simulink model "quadripulse_controller16"  (R2016a)
settings: Solver=FixedStepAuto  StartTime=0.0  StopTime=Inf  RelTol=1e-3
values from neighbouring files (symbols this model uses):
  amplitudeinterval = [0 10000]    [PIP_SetVariables4Compilation.m]
  amplitudeinterval_percentiles = [0.25 0.75]    [PIP_SetVariables4Compilation.m]
  closedloopmode = 0    [PIP_SetVariables4Compilation.m]
  fft_bin_indices_zero_based = [8 13]    [PIP_SetVariables4Compilation.m]
  fir_filter_coefficients = get(design(fdesign.bandpass('n,fst1,fp1,fp2,fst2', 128, 4, 8, 12, 16, 1000), 'firls', 'FilterStructure', 'dffirt'), 'Numerator')    [PIP_SetVariables4Compilation.m]
  forecast_offset_ms = 0    [PIP_SetVariables4Compilation.m]
  marker_id = 0    [PIP_SetVariables4Compilation.m]
  phasecondition = 1    [PIP_SetVariables4Compilation.m]
  reset = 0    [PIP_SetVariables4Compilation.m]
  spatial_filter = zeros(1,N); spatial_filter(chan_center) = 1; spatial_filter(chan_surround) = -1/length(chan_surround)    [PIP_SetVariables4Compilation.m]
  timeinsecondsandtriggerchannel = [0,1;0.1,2]    [PIP_SetVariables4Compilation.m]
undefined symbols (not defined in the file or in its folder): a, b, Columns, MF, PD2, Radix, Rows
libraries: dspmtrx3 x11, slrtlib x10, simulink x9, dspstat3 x5, dspsigops x4, commsequence2 x1, dspobslib x1, dspspect3 x1, dspfdesign x1, xpcueilib x1, xpcparallelportlib x1, xpciplib x1
settings Model: SimulationMode=external  Creator=BNP Lab User  LastModifiedBy=BNP Lab
settings SolverCC: EnableConcurrentExecution=on
settings DataIOCC: LimitDataPoints=on  SaveFormat=StructureWithTime  SaveOutput=off  SignalLogging=off  DSMLogging=off  SaveTime=off
settings OptimizationCC: BlockReduction=off  OptimizeBlockIOStorage=off  BufferReuse=off  GlobalBufferReuse=off  ExpressionFolding=off  LocalBlockOutputs=off
settings DebuggingCC: AllowSymbolicDim=off
settings HardwareCC: ProdBitPerPointer=32  ProdLargestAtomicFloat=None  ProdWordSize=32  ProdHWDeviceType=Generic->32-bit x86 compatible
settings ModelReferenceCC: PropagateSignalLabelsOutOfModel=off
settings RTWCC: SystemTargetFile=slrt.tlc  TemplateMakefile=slrt_default_tmf  Description=Simulink Real-Time  RTWCompilerOptimization=on

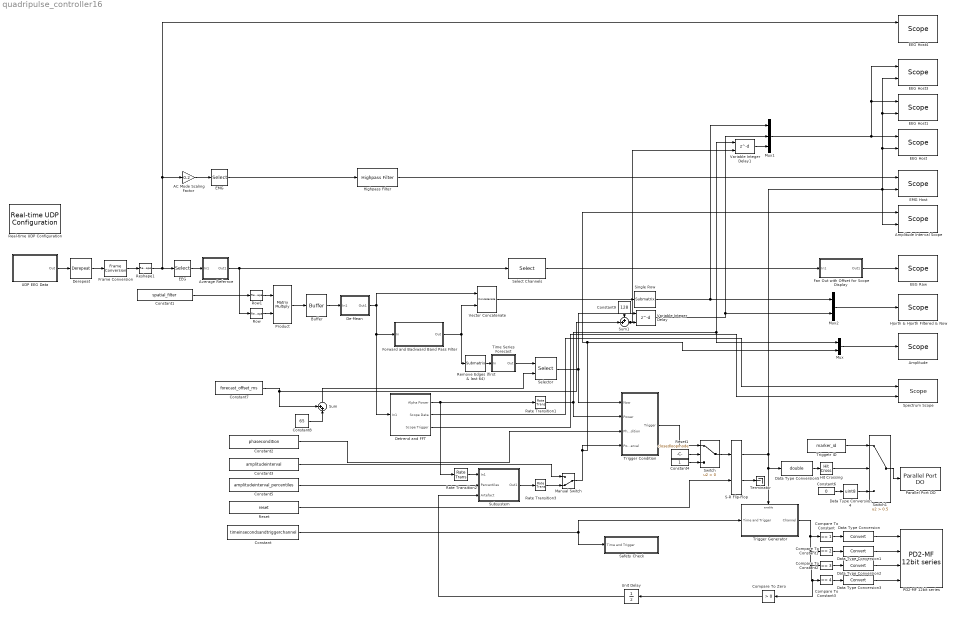
== system quadripulse_controller16 ==
  " Amplitude" : slrtlib/Displays and Logging/Scope   scopeno=3  scopetype=Target  autostart=on  viewmode=Graphical sliding  formatstr='%15.6f'  grid=on  ylimits=[0,0]  nosamples=100  noprepostsamples=0  interleave=100  triggermode=FreeRun  triggersignal=1  trigsignalfromport=on  triggerlevel=0.5  triggerslope=Rising  triggerscope=1  triggersample=0  filename=data.dat  mode=Lazy  writesize=512  autorestart=off  dynamicfilemode=off  maxwritefilesize=512*1024^2
  AC Mode Scaling Factor : Gain  Gain=0.2
  Amplitude Interval Scope : slrtlib/Displays and Logging/Scope   scopeno=10  scopetype=Host  autostart=on  viewmode=Graphical redraw  formatstr='%15.6f'  grid=on  ylimits=[0,0]  nosamples=3  noprepostsamples=-2  interleave=1  triggermode=Signal triggering  triggersignal=1  trigsignalfromport=on  triggerlevel=0.5  triggerslope=Rising  triggerscope=1  triggersample=0  filename=data.dat  mode=Lazy  writesize=512  autorestart=off  dynamicfilemode=off  maxwritefilesize=512*1024^2
  Average Refernce : Subsystem
  Buffer : Buffer  N=512  V=511  TreatMby1Signals=One channel  OutputFrames=off
  Compare To Constant : simulink/Logic and Bit Operations/Compare To Constant  relop===  const=1  OutDataTypeStr=boolean
  Compare To Constant1 : simulink/Logic and Bit Operations/Compare To Constant  relop===  const=2  OutDataTypeStr=boolean
  Compare To Constant2 : simulink/Logic and Bit Operations/Compare To Constant  relop===  const=3  OutDataTypeStr=boolean
  Compare To Constant3 : simulink/Logic and Bit Operations/Compare To Constant  relop===  const=4  OutDataTypeStr=boolean
  Compare To Zero : simulink/Logic and Bit Operations/Compare To Zero  relop=>  OutDataTypeStr=boolean
  Constant : Constant  Value=timeinsecondsandtriggerchannel  OutDataTypeStr=double  SampleTime=-1
  Constant1 : Constant  Value=spatial_filter  SampleTime=-1
  Constant2 : Constant  Value=phasecondition  SampleTime=-1
  Constant3 : Constant  Value=amplitudeinterval  SampleTime=-1
  Constant4 : Constant  OutDataTypeStr=boolean
  Constant5 : Constant  Value=amplitudeinterval_percentiles  SampleTime=-1
  Constant6 : Constant  Value=0  OutDataTypeStr=boolean
  Constant7 : Constant  Value=forecast_offset_ms  SampleTime=-1
  Constant8 : Constant  Value=65
  Constant9 : Constant  Value=128
  Data Type Conversion{,1..3} (4 alike) : DataTypeConversion
  Data Type Conversion4 : DataTypeConversion  OutDataTypeStr=uint8
  Data Type Conversion5 : DataTypeConversion  OutDataTypeStr=double
  De-Mean : Subsystem
  Derepeat : commsequence2/Derepeat  N=5  mode=Unused parameter value  InputProcessing=Columns as channels (frame based)  RateOptions=Enforce single-rate processing  ic=0
  Detrend and FFT : Subsystem
  EEG : Selector  InputPortWidth=66  IndexOptions=Index vector (dialog)  Indices=1:64  OutputSizes=1
  EEG Host : slrtlib/Displays and Logging/Scope   scopeno=12  scopetype=Host  autostart=on  viewmode=Graphical redraw  formatstr='%15.6f'  grid=on  ylimits=[0,0]  nosamples=3000  noprepostsamples=-3000  interleave=1  triggermode=Signal triggering  triggersignal=1  trigsignalfromport=on  triggerlevel=0.5  triggerslope=Rising  triggerscope=1  triggersample=0  filename=data.dat  mode=Lazy  writesize=512  autorestart=off  dynamicfilemode=off  maxwritefilesize=512*1024^2
  EEG Host1 : slrtlib/Displays and Logging/Scope   scopeno=13  scopetype=Host  autostart=on  viewmode=Graphical redraw  formatstr='%15.6f'  grid=on  ylimits=[0,0]  nosamples=2000  noprepostsamples=-1000+128  interleave=1  triggermode=Signal triggering  triggersignal=1  trigsignalfromport=on  triggerlevel=0.5  triggerslope=Rising  triggerscope=1  triggersample=0  filename=data.dat  mode=Lazy  writesize=512  autorestart=off  dynamicfilemode=off  maxwritefilesize=512*1024^2
  EEG Host3 : slrtlib/Displays and Logging/Scope   scopeno=14  scopetype=Host  autostart=on  viewmode=Graphical redraw  formatstr='%15.6f'  grid=on  ylimits=[0,0]  nosamples=150  noprepostsamples=-50+128  interleave=1  triggermode=Signal triggering  triggersignal=1  trigsignalfromport=on  triggerlevel=0.5  triggerslope=Rising  triggerscope=1  triggersample=0  filename=data.dat  mode=Lazy  writesize=512  autorestart=off  dynamicfilemode=off  maxwritefilesize=512*1024^2
  EEG Host4 : slrtlib/Displays and Logging/Scope   scopeno=15  scopetype=Host  autostart=on  viewmode=Graphical redraw  formatstr='%15.6f'  grid=on  ylimits=[0,0]  nosamples=2000  noprepostsamples=-1000  interleave=1  triggermode=Signal triggering  triggersignal=1  trigsignalfromport=on  triggerlevel=0.5  triggerslope=Rising  triggerscope=1  triggersample=0  filename=data.dat  mode=Lazy  writesize=512  autorestart=off  dynamicfilemode=off  maxwritefilesize=512*1024^2
  EEG Raw : slrtlib/Displays and Logging/Scope   scopeno=1  scopetype=Target  autostart=on  viewmode=Graphical redraw  formatstr='%15.6f'  grid=on  ylimits=[0,0]  nosamples=500  noprepostsamples=-250  interleave=1  triggermode=FreeRun  triggersignal=1  trigsignalfromport=on  triggerlevel=0.5  triggerslope=Rising  triggerscope=1  triggersample=0  filename=data.dat  mode=Lazy  writesize=512  autorestart=off  dynamicfilemode=off  maxwritefilesize=512*1024^2
  EMG : Selector  InputPortWidth=66  IndexOptions=Index vector (dialog)  Indices=[65 66]  OutputSizes=1
  "EMG Host " : slrtlib/Displays and Logging/Scope   scopeno=11  scopetype=Host  autostart=on  viewmode=Graphical redraw  formatstr='%15.6f'  grid=on  ylimits=[0,0]  nosamples=150  noprepostsamples=50  interleave=1  triggermode=Signal triggering  triggersignal=1  trigsignalfromport=on  triggerlevel=0.5  triggerslope=Rising  triggerscope=1  triggersample=0  filename=data.dat  mode=Lazy  writesize=512  autorestart=off  dynamicfilemode=off  maxwritefilesize=512*1024^2
  "Fan Out with Offset for Scope Display " : Subsystem
  Forward and Backward Band Pass Filter : Subsystem
  Frame Conversion : FrameConversion  InheritSamplingMode=off  OutFrame=Sample-based
  Highpass Filter : dspfdesign/Highpass Filter  FilterType=FIR  DesignForMinimumOrder=off  FilterOrder=200  StopbandFrequency=8e3  PassbandFrequency=10  StopbandAttenuation=80  PassbandRipple=0.1  InheritSampleRate=off  SampleRate=1000  roundingMode=Floor  coeffsDataTypeStr=fixdt(1,16)  SimulateUsing=Interpreted execution
  Hit Crossing : HitCross  HitCrossingOffset=0.5  HitCrossingDirection=rising
  Hjorth & Hjorth Filtered & Now : slrtlib/Displays and Logging/Scope   scopeno=2  scopetype=Target  autostart=on  viewmode=Graphical redraw  formatstr='%15.6f'  grid=on  ylimits=[-0,0]  nosamples=500  noprepostsamples=-250+128  interleave=1  triggermode=FreeRun  triggersignal=1  trigsignalfromport=on  triggerlevel=0.5  triggerslope=Rising  triggerscope=1  triggersample=0  filename=data.dat  mode=Lazy  writesize=512  autorestart=off  dynamicfilemode=off  maxwritefilesize=512*1024^2
  Manual Switch : ManualSwitch  CurrentSetting=0
  Mux : Mux  Inputs=2
  Mux1 : Mux  Inputs=3
  Mux2 : Mux  Inputs=2
  PD2-MF 12bit series : xpcueilib/Digital Output/PD2-MF 12bit series  boardtypein=PD2-MF-64-3M/12H  channel=[1 2 3 4]  reset=[1 1 1 1]  initValue=[0 0 0 0]  sampletime=0.001  pcislot=-1
  "Parallel Port DO " : xpcparallelportlib/Digital Output/Parallel Port DO   BaseMask=Other  BaseString=0xc010  Format=Single 8-bit Port  Channels=[1]  InitialValues=[0]  FinalActions=[0]  FinalValues=[0]  SampleTime=0.001  Mode=1
  Product : Product  Multiplication=Matrix(*)
  Rate Transition1 : RateTransition  Integrity=off  OutPortSampleTimeOpt=Inherit  OutPortSampleTime=10
  Rate Transition2 : RateTransition  Integrity=off  OutPortSampleTime=0.1
  Rate Transition3 : RateTransition  Integrity=off  OutPortSampleTimeOpt=Inherit  OutPortSampleTime=0.1
  Real-time UDP Configuration : xpciplib/Real-time UDP  Configuration   ID=1  IpAddress=192.168.200.240  SubnetMask=255.255.255.0  Gateway=0.0.0.0  EthDrv=Intel Gigabit  PciBus=3  PciSlot=0  udpID=0  MulticastList=[]  Multicast={}
  Remove Edges (first & last 64) : dspmtrx3/Submatrix  RowSpan=Range of rows  RowStartMode=Index  RowStartIndex=65  RowEndMode=Offset from last  RowEndIndex=64  ColSpan=All columns  ColStartMode=First  ColStartIndex=1  ColEndMode=Offset from last  ColEndIndex=20
  Reset : Constant  Value=reset  OutDataTypeStr=boolean  SampleTime=0.001
  Reset1 : Constant  Value=closedloopmode  OutDataTypeStr=boolean  SampleTime=0.001
  Reshape1 : Reshape  OutputDimensionality=Row vector (2-D)
  Row : Reshape  OutputDimensionality=Column vector (2-D)
  Row1 : Reshape  OutputDimensionality=Row vector (2-D)
  S-R Flip-Flop : simulink_extras/Flip Flops/S-R Flip-Flop  initial_condition=0
  Safety Check : Subsystem
  Select Channels : Selector  InputPortWidth=65  IndexOptions=Index vector (dialog)  Indices=[5 21 23 25 27]  OutputSizes=1
  Selector : Selector  InputPortWidth=128  IndexOptions=Index vector (port)  Indices=forecast_offset_ms  OutputSizes=1
  Single Row : dspmtrx3/Submatrix  RowSpan=One row  RowStartMode=Offset from last  RowStartIndex=128  RowEndMode=Last  RowEndIndex=1  ColSpan=All columns  ColStartMode=Index  ColStartIndex=1  ColEndMode=Last  ColEndIndex=1
  "Spectrum Scope " : slrtlib/Displays and Logging/Scope   scopeno=4  scopetype=Target  autostart=on  viewmode=Graphical redraw  formatstr='%15.6f'  grid=on  ylimits=[0,0]  nosamples=100  noprepostsamples=0  interleave=1  triggermode=Signal triggering  triggersignal=1  trigsignalfromport=on  triggerlevel=0.5  triggerslope=Rising  triggerscope=1  triggersample=0  filename=data.dat  mode=Lazy  writesize=512  autorestart=off  dynamicfilemode=off  maxwritefilesize=512*1024^2
  Subsystem : Subsystem
  Sum : Sum  Inputs=++|
  Sum1 : Sum  Inputs=++|
  Switch : Switch  Criteria=u2 > Threshold
  Switch1 : Switch  Criteria=u2 > Threshold  Threshold=0.5
  Terminator : Terminator
  Time Series Forecast : Subsystem
  Trigger Condition : Subsystem
  Trigger Generator : Subsystem
  Triggetr ID : Constant  Value=marker_id  OutDataTypeStr=uint8  SampleTime=0.001
  UDP EEG Data : Subsystem  mask{chans=66, frame=5, recordingMode=DC}
      mask prompts: chans "Number of channels"; frame "Samples per packet"; recordingMode "Recording Mode:"
      mask init:
      | scalingFactor = 50; %default scaling factor (AC mode)
      | blk = gcb;
      | recordingModeString = get_param(blk,'recordingMode');
      | if strcmp(recordingModeString, 'DC')
      |     scalingFactor = 10;
      | end
      mask TypeOptions recordingMode: AC | DC
  Unit Delay : UnitDelay  SampleTime=-1
  Variable Integer Delay : Delay  DelayLengthSource=Input port  DelayLengthUpperLimit=128+63
      settings: InputPortMap=u0,p1
  Variable Integer Delay1 : Delay  DelayLengthSource=Input port  DelayLengthUpperLimit=128+63
      settings: InputPortMap=u0,p1
  Vector Concatenate : Concatenate  Mode=Multidimensional array  ConcatenateDimension=2
  wires:
  Compare To Constant/1 -> Data Type Conversion/1
  Compare To Constant1/1 -> Data Type Conversion1/1
  Compare To Constant2/1 -> Data Type Conversion2/1
  Compare To Constant3/1 -> Data Type Conversion3/1
  Data Type Conversion2/1 -> PD2-MF 12bit series/3
  Data Type Conversion3/1 -> PD2-MF 12bit series/4
  EMG/1 -> Highpass Filter/1
  "Fan Out with Offset for Scope Display "/1(Out1) -> EEG Raw/1
  Reshape1/1 -> AC Mode Scaling Factor/1, EEG Host4/1, EEG/1
  Vector Concatenate/1 -> Single Row/1
  Buffer/1 -> De-Mean/1(In1)
  Forward and Backward Band Pass Filter/1(Out) -> Vector Concatenate/2, Remove Edges (first & last 64)/1
  Remove Edges (first & last 64)/1 -> Time Series Forecast/1(In)
  Time Series Forecast/1(Out) -> Selector/1
  Detrend and FFT/1(Alpha Power) -> Rate Transition2/1, Rate Transition1/1
  Trigger Generator/1(Channel) -> Compare To Zero/1, Compare To Constant3/1, Compare To Constant2/1, Compare To Constant1/1, Compare To Constant/1
  Constant/1 -> Trigger Generator/1(Time and Trigger), Safety Check/1(Time and Trigger)
  Reset/1 -> S-R Flip-Flop/2
  S-R Flip-Flop/2 -> Terminator/1
  S-R Flip-Flop/1 -> Amplitude Interval Scope/2, EEG Host3/2, EEG Host1/2, EEG Host/2, "EMG Host "/2, Trigger Generator/Enable, Data Type Conversion5/1
  Trigger Condition/1(Trigger) -> Switch/1
  Switch/1 -> S-R Flip-Flop/1
  Reset1/1 -> Switch/2
  Constant4/1 -> Switch/3
  Constant2/1 -> Trigger Condition/3(Phase Condition)
  Switch1/1 -> "Parallel Port DO "/1
  Mux1/1 -> EEG Host3/1, EEG Host1/1, EEG Host/1
  Single Row/1 -> Mux1/1, Mux2/1
  Data Type Conversion1/1 -> PD2-MF 12bit series/2
  Data Type Conversion/1 -> PD2-MF 12bit series/1
  Mux2/1 -> Hjorth & Hjorth Filtered & Now/1
  Triggetr ID/1 -> Switch1/1
  Constant6/1 -> Data Type Conversion4/1
  Data Type Conversion4/1 -> Switch1/3
  Detrend and FFT/3(Scope Trigger) -> "Spectrum Scope "/2
  Data Type Conversion5/1 -> Hit Crossing/1
  Hit Crossing/1 -> Switch1/2
  UDP EEG Data/1(Out) -> Derepeat/1
  Selector/1 -> Variable Integer Delay/1, Trigger Condition/1(Now)
  Variable Integer Delay1/1 -> Mux1/3
  Derepeat/1 -> Frame Conversion/1
  Row/1 -> Product/2
  Row1/1 -> Product/1
  EEG/1 -> Average Refernce/1(In1)
  Constant1/1 -> Row1/1
  Product/1 -> Buffer/1
  Frame Conversion/1 -> Reshape1/1
  AC Mode Scaling Factor/1 -> EMG/1
  Detrend and FFT/2(Scope Data) -> "Spectrum Scope "/1
  Average Refernce/1(Out1) -> Row/1, Select Channels/1
  Select Channels/1 -> "Fan Out with Offset for Scope Display "/1(In1)
  De-Mean/1(Out1) -> Detrend and FFT/1(In1), Forward and Backward Band Pass Filter/1(In), Vector Concatenate/1
  Variable Integer Delay/1 -> Mux1/2, Mux2/2
  Rate Transition1/1 -> Variable Integer Delay1/1, Mux/1, Trigger Condition/2(Power)
  Rate Transition2/1 -> Subsystem/1(In1)
  Subsystem/1(Out1) -> Rate Transition3/1
  Constant3/1 -> Manual Switch/1
  Manual Switch/1 -> Amplitude Interval Scope/1, Mux/2, Trigger Condition/4(Power Interval)
  Rate Transition3/1 -> Manual Switch/2
  Constant5/1 -> Subsystem/2(Percentiles)
  Compare To Zero/1 -> Unit Delay/1
  Unit Delay/1 -> Subsystem/3(Artefact)
  Mux/1 -> " Amplitude"/1
  Highpass Filter/1 -> "EMG Host "/1
  Constant7/1 -> Sum/1, Sum1/2
  Sum/1 -> Selector/2
  Constant8/1 -> Sum/2
  Sum1/1 -> Variable Integer Delay1/2, Variable Integer Delay/2
  Constant9/1 -> Sum1/1

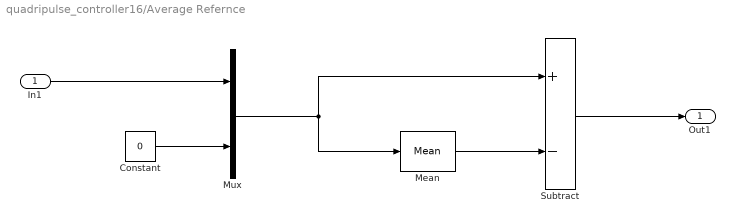
== system quadripulse_controller16/Average Refernce ==
  In1 : Inport
  Constant : Constant  Value=0
  Mean : dspstat3/Mean  run=off  reset_popup=None  InputProcessing=Columns as channels (frame based)  directionMode=Entire input  dimension=1  roiEnable=off  roiType=Rectangles  roiPortion=Entire ROI  roiOutput=Individual statistics for each ROI  roiFlag=off  outputDataTypeStr=Inherit: Same as accumulator  outputLastDataTypeStr=Inherit: Same as accumulator  outputMin=[]  outputMax=[]  roundingMode=Floor  overflowMode=off
  Mux : Mux  Inputs=2
  Subtract : Sum  Inputs=+-
  Out1 : Outport
  wires:
  Mean/1 -> Subtract/2
  Constant/1 -> Mux/2
  In1/1 -> Mux/1
  Mux/1 -> Subtract/1, Mean/1
  Subtract/1 -> Out1/1

== system quadripulse_controller16/De-Mean ==
  In1 : Inport
  Mean : dspstat3/Mean  run=off  reset_popup=None  InputProcessing=Columns as channels (frame based)  directionMode=Entire input  dimension=1  roiEnable=off  roiType=Rectangles  roiPortion=Entire ROI  roiOutput=Individual statistics for each ROI  roiFlag=off  outputDataTypeStr=Inherit: Same as accumulator  outputLastDataTypeStr=Inherit: Same as accumulator  outputMin=[]  outputMax=[]  roundingMode=Floor  overflowMode=off
  Subtract : Sum  Inputs=+-
  Out1 : Outport
  wires:
  Subtract/1 -> Out1/1
  Mean/1 -> Subtract/2
  In1/1 -> Subtract/1, Mean/1

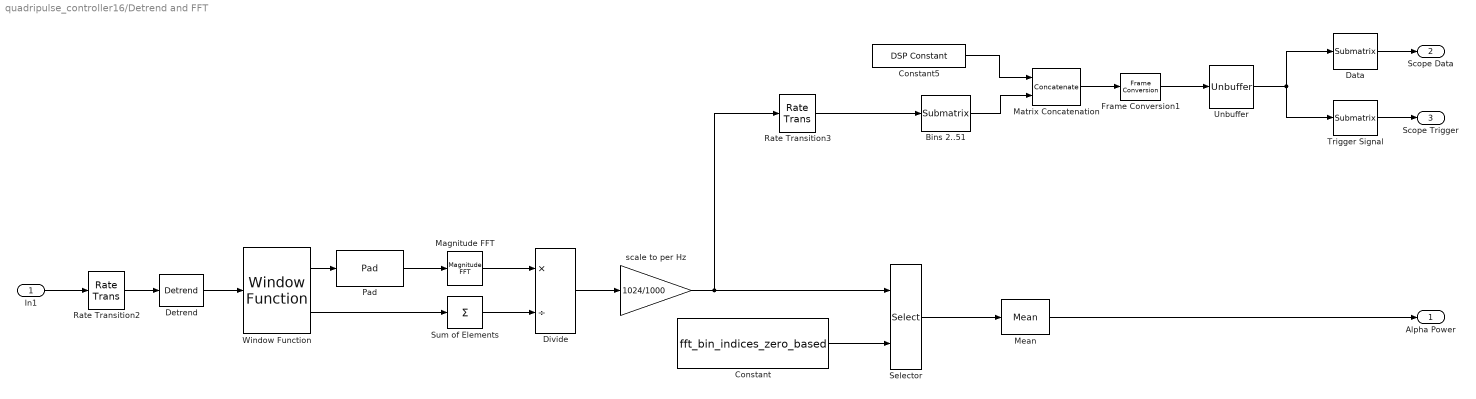
== system quadripulse_controller16/Detrend and FFT ==
  In1 : Inport
  Bins 2..51 : dspmtrx3/Submatrix  RowSpan=Range of rows  RowStartMode=Index  RowStartIndex=2  RowEndMode=Index  RowEndIndex=101  ColSpan=All columns  ColStartMode=First  ColStartIndex=1  ColEndMode=Last  ColEndIndex=1
  Constant : Constant  Value=fft_bin_indices_zero_based  SampleTime=-1
  Constant5 : dspobslib/DSP Constant  Value=[0.5;zeros(100-1,1)]  SampleMode=Discrete  discreteOutput=Sample-based  continuousOutput=Sample-based  sampTime=-1  framePeriod=-1  dataType=Inherit from 'Constant value'  isSigned=on  wordLen=16  udDataType=sfix(16)  fracBitsMode=Best precision  numFracBits=15  InterpretAs1D=off  Ts=-1  FramebasedOutput=off
  Data : dspmtrx3/Submatrix  RowSpan=All rows  RowStartMode=First  RowStartIndex=1  RowEndMode=Last  RowEndIndex=1  ColSpan=Range of columns  ColStartMode=Index  ColStartIndex=2  ColEndMode=Last  ColEndIndex=1
  Detrend : dspstat3/Detrend
  Divide : Product  Inputs=*/
  Frame Conversion1 : FrameConversion  InheritSamplingMode=off
  Magnitude FFT : dspspect3/Magnitude FFT  mag_or_magsq=Magnitude squared  FFTImplementation=Radix-2  fftLenInherit=on  fftsize=256  WrapInput=on
  Matrix Concatenation : Concatenate  Mode=Multidimensional array  ConcatenateDimension=2
  Mean : dspstat3/Mean  run=off  reset_popup=None  InputProcessing=Columns as channels (frame based)  directionMode=Entire input  dimension=1  roiEnable=off  roiType=Rectangles  roiPortion=Entire ROI  roiOutput=Individual statistics for each ROI  roiFlag=off  outputDataTypeStr=Inherit: Same as accumulator  outputLastDataTypeStr=Inherit: Same as accumulator  outputMin=[]  outputMax=[]  roundingMode=Floor  overflowMode=off
  Pad : dspsigops/Pad  padAlong=Columns  dimsToPad=1  valSrc=Specify via dialog  padVal=0  spec=Output size  padNumOutRowsSpecMethod=User-specified  numOutRows=1024  padNumOutColsSpecMethod=User-specified  numOutCols=1024  isVarDimsMode=off  padBeginning=0  padEnd=0  outSizeMode=User-specified  outSize=1  padSigAt=Beginning and end  trunc_flag=Error  roundingMode=Floor  overflowMode=off  truncOrWrapMode=Truncate  wrap_flag=None
  Rate Transition2 : RateTransition  Integrity=off  OutPortSampleTime=0.01
  Rate Transition3 : RateTransition  Integrity=off  OutPortSampleTime=0.1
  Selector : Selector  IndexMode=Zero-based  InputPortWidth=1024  IndexOptions=Starting and ending indices (port)  Indices=fft_bin_indices_zero_based  OutputSizes=1
  Sum of Elements : Sum  Inputs=+
  Trigger Signal : dspmtrx3/Submatrix  RowSpan=All rows  RowStartMode=First  RowStartIndex=1  RowEndMode=Last  RowEndIndex=1  ColSpan=One column  ColStartMode=First  ColStartIndex=1  ColEndMode=Last  ColEndIndex=1
  Unbuffer : Unbuffer  SampleBasedProcessing=Same as frame based
  Window Function : dspsigops/Window Function  winmode=Generate and apply window  wintype=Hanning  sampmode=Continuous  samptime=1  N=64  Rs=50  beta=10  winsamp=Symmetric  UserWindow=hamming  OptParams=off  UserParams={'symmetric'}  dataType=double  isSigned=on  wordLen=16  udDataType=sfix(16)  fracBitsMode=Best precision  numFracBits=15  roundingMode=Floor  overflowMode=off  numSidelobes=4  sidelobeLevel=-30
  scale to per Hz : Gain  Gain=1024/1000
  Alpha Power : Outport
  Scope Data : Outport  Port=2
  Scope Trigger : Outport  Port=3
  wires:
  Mean/1 -> Alpha Power/1
  Selector/1 -> Mean/1
  In1/1 -> Rate Transition2/1
  Divide/1 -> scale to per Hz/1
  Rate Transition2/1 -> Detrend/1
  Window Function/2 -> Sum of Elements/1
  Sum of Elements/1 -> Divide/2
  Window Function/1 -> Pad/1
  Magnitude FFT/1 -> Divide/1
  scale to per Hz/1 -> Selector/1, Rate Transition3/1
  Frame Conversion1/1 -> Unbuffer/1
  Unbuffer/1 -> Trigger Signal/1, Data/1
  Constant5/1 -> Matrix Concatenation/1
  Bins 2..51/1 -> Matrix Concatenation/2
  Matrix Concatenation/1 -> Frame Conversion1/1
  Data/1 -> Scope Data/1
  Trigger Signal/1 -> Scope Trigger/1
  Rate Transition3/1 -> Bins 2..51/1
  Pad/1 -> Magnitude FFT/1
  Detrend/1 -> Window Function/1
  Constant/1 -> Selector/2

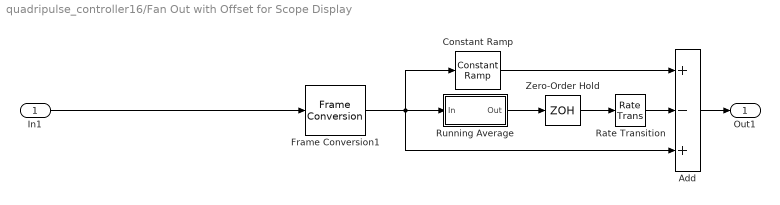
== system quadripulse_controller16/Fan Out with Offset for Scope Display  ==
  In1 : Inport
  Add : Sum  Inputs=+-+
  Constant Ramp : dspsigops/Constant Ramp  L=Columns  dim=2  Slope=5  dataType=Same as input  isSigned=on  wordLen=16  udDataType=sfix(16)  fracBitsMode=Best precision  numFracBits=15  Offset=0
  Frame Conversion1 : FrameConversion  InheritSamplingMode=off  OutFrame=Sample-based
  Rate Transition : RateTransition  Integrity=off  OutPortSampleTimeOpt=Inherit  OutPortSampleTime=0.5
  Running Average : Subsystem  mask{N=500}
      mask prompts: N "Delay in Time Steps"
  Zero-Order Hold : ZeroOrderHold  SampleTime=0.5
  Out1 : Outport
  wires:
  In1/1 -> Frame Conversion1/1
  Rate Transition/1 -> Add/2
  Zero-Order Hold/1 -> Rate Transition/1
  Frame Conversion1/1 -> Constant Ramp/1, Add/3, Running Average/1(In)
  Running Average/1(Out) -> Zero-Order Hold/1
  Constant Ramp/1 -> Add/1
  Add/1 -> Out1/1

== system quadripulse_controller16/Forward and Backward Band Pass Filter ==
  In : Inport
  FIR Bandpass Filter Backward : DiscreteFir  Tag=BlockMethodSubSystem  Coefficients=fir_filter_coefficients  InputProcessing=Columns as channels (frame based)
  FIR Bandpass Filter Forward : DiscreteFir  Tag=BlockMethodSubSystem  Coefficients=fir_filter_coefficients  InputProcessing=Columns as channels (frame based)
  Flip : DSPFlip
  Re-Flip : DSPFlip
  Out : Outport
  wires:
  In/1 -> FIR Bandpass Filter Forward/1
  Re-Flip/1 -> Out/1
  FIR Bandpass Filter Backward/1 -> Re-Flip/1
  FIR Bandpass Filter Forward/1 -> Flip/1
  Flip/1 -> FIR Bandpass Filter Backward/1

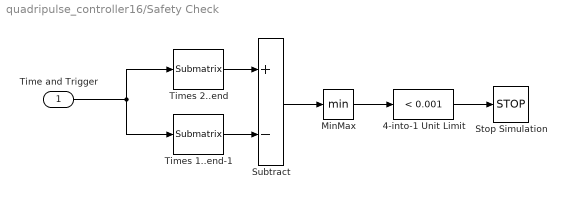
== system quadripulse_controller16/Safety Check ==
  Time and Trigger : Inport
  4-into-1 Unit Limit : simulink/Logic and Bit Operations/Compare To Constant  relop=<  const=0.001  OutDataTypeStr=boolean
  MinMax : MinMax
  Stop Simulation : Stop
  Subtract : Sum  Inputs=+-
  Times 1..end-1 : dspmtrx3/Submatrix  RowSpan=Range of rows  RowStartMode=First  RowStartIndex=1  RowEndMode=Offset from last  RowEndIndex=1  ColSpan=One column  ColStartMode=First  ColStartIndex=1  ColEndMode=Last  ColEndIndex=1
  Times 2..end : dspmtrx3/Submatrix  RowSpan=Range of rows  RowStartMode=Index  RowStartIndex=2  RowEndMode=Last  RowEndIndex=1  ColSpan=One column  ColStartMode=First  ColStartIndex=1  ColEndMode=Last  ColEndIndex=1
  wires:
  MinMax/1 -> 4-into-1 Unit Limit/1
  Times 2..end/1 -> Subtract/1
  4-into-1 Unit Limit/1 -> Stop Simulation/1
  Subtract/1 -> MinMax/1
  Times 1..end-1/1 -> Subtract/2
  Time and Trigger/1 -> Times 2..end/1, Times 1..end-1/1

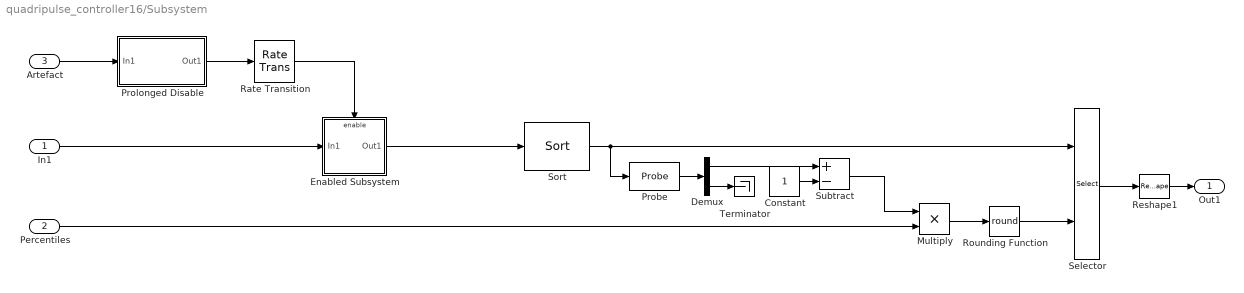
== system quadripulse_controller16/Subsystem ==
  In1 : Inport
  Percentiles : Inport  Port=2
  Artefact : Inport  Port=3
  Constant : Constant
  Demux : Demux  Outputs=2
  Enabled Subsystem : Subsystem  TreatAsAtomicUnit=on
  Multiply : Product  Inputs=**
  Probe : Probe  ProbeWidth=off  ProbeSampleTime=off  ProbeComplexSignal=off  ProbeSignalDimensions=on
  Prolonged Disable : Subsystem
  Rate Transition : RateTransition
  Reshape1 : Reshape
  Rounding Function : Rounding  Operator=round
  Selector : Selector  IndexMode=Zero-based  InputPortWidth=600  IndexOptions=Index vector (port)  Indices=[a b]  OutputSizes=1
  Sort : dspstat3/Sort  otype=Value  dir=Ascending  sortAlg=Quick sort  accumDataTypeStr=Inherit: Same as product output  accumLastDataTypeStr=Inherit: Same as product output  roundingMode=Floor  overflowMode=off
  Subtract : Sum  Inputs=+-
  Terminator : Terminator
  Out1 : Outport
  wires:
  Sort/1 -> Probe/1, Selector/1
  Selector/1 -> Reshape1/1
  Percentiles/1 -> Multiply/2
  Rounding Function/1 -> Selector/2
  Probe/1 -> Demux/1
  Demux/1 -> Subtract/1
  Multiply/1 -> Rounding Function/1
  Demux/2 -> Terminator/1
  Constant/1 -> Subtract/2
  Subtract/1 -> Multiply/1
  In1/1 -> Enabled Subsystem/1(In1)
  Rate Transition/1 -> Enabled Subsystem/Enable
  Artefact/1 -> Prolonged Disable/1(In1)
  Prolonged Disable/1(Out1) -> Rate Transition/1
  Enabled Subsystem/1(Out1) -> Sort/1
  Reshape1/1 -> Out1/1

== system quadripulse_controller16/Time Series Forecast ==
  In : Inport
  Forecast of 128 samples : Subsystem  mask{num_iterations=128}
      mask prompts: num_iterations "Number of iterations (number of predicted samples)"
  Frame Conversion : FrameConversion  InheritSamplingMode=off
  Terminator : Terminator
  Yule-Walker AR Estimator : dspparest3/Yule-Walker AR Estimator  ywArOutType=A  inheritOrder=off  ord=30
  Out : Outport
  wires:
  Forecast of 128 samples/1(Out1) -> Out/1
  Yule-Walker AR Estimator/1 -> Forecast of 128 samples/2(Coefficients)
  Yule-Walker AR Estimator/2 -> Terminator/1
  Frame Conversion/1 -> Yule-Walker AR Estimator/1
  In/1 -> Frame Conversion/1, Forecast of 128 samples/1(Data)

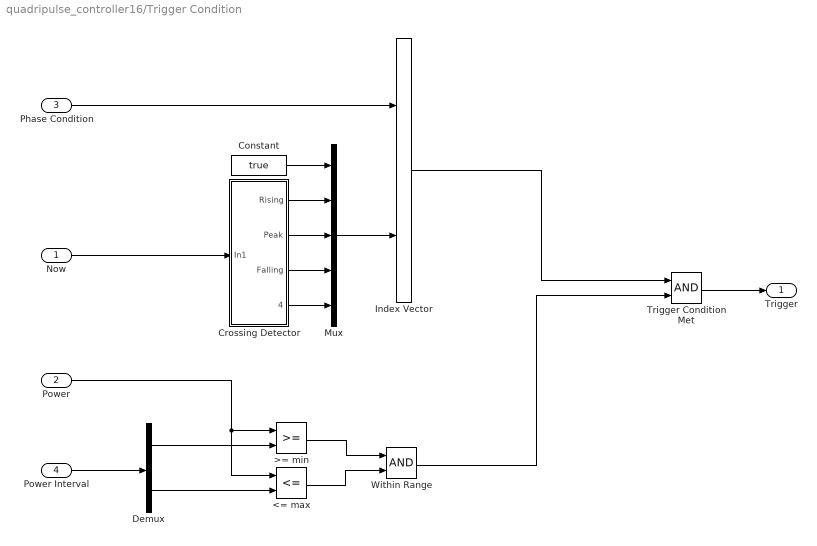
== system quadripulse_controller16/Trigger Condition ==
  Now : Inport
  Power : Inport  Port=2
  Phase Condition : Inport  Port=3
  Power Interval : Inport  Port=4  PortDimensions=2
  <= max : RelationalOperator  Operator=<=  OutDataTypeStr=boolean
  >= min : RelationalOperator  OutDataTypeStr=boolean
  Constant : Constant  Value=true
  Crossing Detector : Subsystem
  Demux : Demux  Outputs=2
  Index Vector : MultiPortSwitch  DataPortOrder=Zero-based contiguous  Inputs=1
  Mux : Mux  Inputs=5
  Trigger Condition Met : Logic  AllPortsSameDT=off  OutDataTypeStr=boolean
  Within Range : Logic  AllPortsSameDT=off  OutDataTypeStr=boolean
  Trigger : Outport
  wires:
  Mux/1 -> Index Vector/2
  Phase Condition/1 -> Index Vector/1
  Index Vector/1 -> Trigger Condition Met/1
  Power Interval/1 -> Demux/1
  Demux/1 -> >= min/2
  Power/1 -> <= max/1, >= min/1
  Demux/2 -> <= max/2
  >= min/1 -> Within Range/1
  <= max/1 -> Within Range/2
  Within Range/1 -> Trigger Condition Met/2
  Trigger Condition Met/1 -> Trigger/1
  Now/1 -> Crossing Detector/1(In1)
  Crossing Detector/1(Rising) -> Mux/2
  Crossing Detector/2(Peak) -> Mux/3
  Crossing Detector/3(Falling) -> Mux/4
  Crossing Detector/4(Trough) -> Mux/5
  Constant/1 -> Mux/1

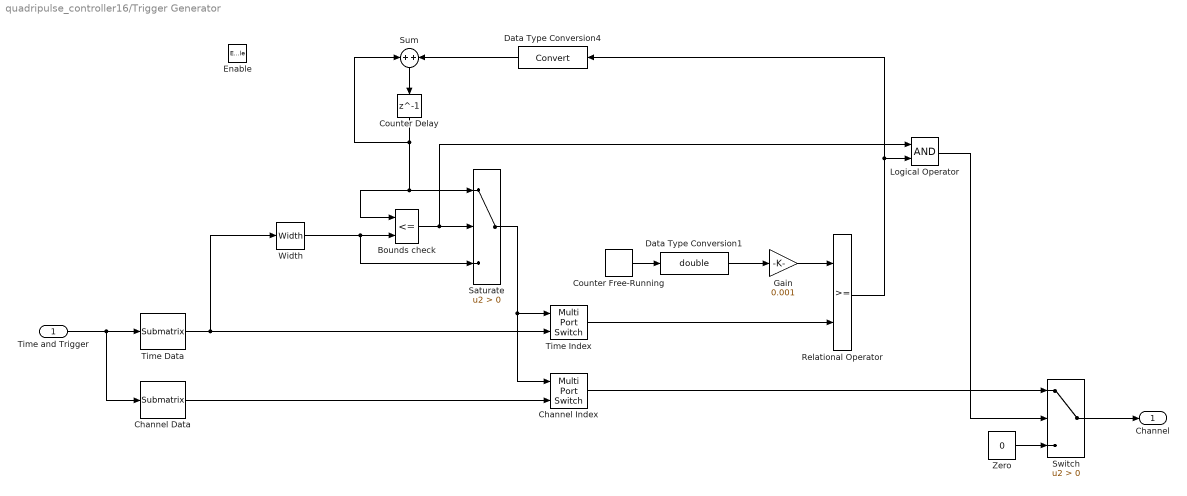
== system quadripulse_controller16/Trigger Generator ==
  Time and Trigger : Inport
  Enable : EnablePort  StatesWhenEnabling=reset
  Bounds check : RelationalOperator  Operator=<=  OutDataTypeStr=boolean
  Channel Data : dspmtrx3/Submatrix  RowSpan=All rows  RowStartMode=First  RowStartIndex=1  RowEndMode=Last  RowEndIndex=1  ColSpan=One column  ColStartMode=Last  ColStartIndex=1  ColEndMode=Last  ColEndIndex=1
  Channel Index : MultiPortSwitch  Inputs=1
  Counter Free-Running : simulink/Sources/Counter Free-Running  NumBits=32  tsamp=-1
  Counter Delay : Delay  DelayLength=1  InitialCondition=1
  Data Type Conversion1 : DataTypeConversion  OutDataTypeStr=double
  Data Type Conversion4 : DataTypeConversion
  Gain : Gain  Gain=0.001
  Logical Operator : Logic  AllPortsSameDT=off  OutDataTypeStr=boolean
  Relational Operator : RelationalOperator  OutDataTypeStr=boolean
  Saturate : Switch  Criteria=u2 > Threshold
  Sum : Sum  Inputs=+|+  AccumDataTypeStr=uint32
  Switch : Switch  Criteria=u2 > Threshold
  Time Data : dspmtrx3/Submatrix  RowSpan=All rows  RowStartMode=First  RowStartIndex=1  RowEndMode=Last  RowEndIndex=1  ColSpan=One column  ColStartMode=First  ColStartIndex=1  ColEndMode=Last  ColEndIndex=1
  Time Index : MultiPortSwitch  Inputs=1
  Width : Width
  Zero : Constant  Value=0
  Channel : Outport
  wires:
  Switch/1 -> Channel/1
  Time and Trigger/1 -> Channel Data/1, Time Data/1
  Relational Operator/1 -> Logical Operator/2, Data Type Conversion4/1
  Time Index/1 -> Relational Operator/2
  Gain/1 -> Relational Operator/1
  Sum/1 -> Counter Delay/1
  Time Data/1 -> Width/1, Time Index/2
  Channel Index/1 -> Switch/1
  Zero/1 -> Switch/3
  Channel Data/1 -> Channel Index/2
  Bounds check/1 -> Logical Operator/1, Saturate/2
  Width/1 -> Saturate/3, Bounds check/2
  Counter Delay/1 -> Sum/1, Bounds check/1, Saturate/1
  Saturate/1 -> Channel Index/1, Time Index/1
  Data Type Conversion4/1 -> Sum/2
  Logical Operator/1 -> Switch/2
  Data Type Conversion1/1 -> Gain/1
  Counter Free-Running/1 -> Data Type Conversion1/1

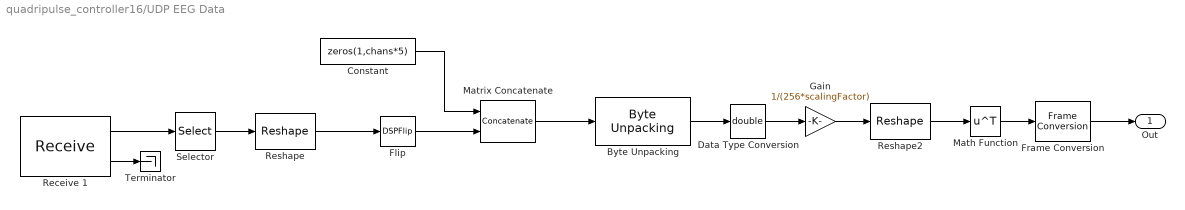
== system quadripulse_controller16/UDP EEG Data ==
  "Byte Unpacking " : xpcutilitieslib/Byte Unpacking   MaskUnpackedDataTypes={'int32'}  MaskUnpackedDataSizes={[chans*5]}  MaskAlignment=1
  Constant : Constant  Value=zeros(1,chans*5)  VectorParams1D=off  OutDataTypeStr=uint8
  Data Type Conversion : DataTypeConversion  OutDataTypeStr=double
  Flip : DSPFlip
  Frame Conversion : FrameConversion  InheritSamplingMode=off
  Gain : Gain  Gain=1/(256*scalingFactor)
  Math Function : Math  Operator=transpose  OutputSignalType=real  SaturateOnIntegerOverflow=on
  Matrix Concatenate : Concatenate  Mode=Multidimensional array
  Receive 1 : xpcrtudplib/Receive   ID=1  Receive1=0.0.0.0  Receive2=50000  Receive3=28+(chans*5*3)  Receive4=0.001  udpID=0
      link override Buffer 1: BufferSize=1
  Reshape : Reshape  OutputDimensionality=Customize  OutputDimensions=[3,chans*5]
  Reshape2 : Reshape  OutputDimensionality=Customize  OutputDimensions=[chans,5]
  Selector : Selector  IndexOptions=Index vector (dialog)  Indices=[29:(29+chans*5*3-1)]  OutputSizes=1
  Terminator : Terminator
  Out : Outport  Unit=uV
  wires:
  Gain/1 -> Reshape2/1
  Frame Conversion/1 -> Out/1
  Receive 1/1 -> Selector/1
  Selector/1 -> Reshape/1
  Receive 1/2 -> Terminator/1
  Constant/1 -> Matrix Concatenate/1
  Matrix Concatenate/1 -> "Byte Unpacking "/1
  "Byte Unpacking "/1 -> Data Type Conversion/1
  Data Type Conversion/1 -> Gain/1
  Reshape/1 -> Flip/1
  Flip/1 -> Matrix Concatenate/2
  Reshape2/1 -> Math Function/1
  Math Function/1 -> Frame Conversion/1

== system quadripulse_controller16/Fan Out with Offset for Scope Display /Running Average ==
  In : Inport
  Add : Sum  Inputs=++-
  Delay : Delay  DelayLength=N  InitialCondition=0  InputProcessing=Columns as channels (frame based)  UseCircularBuffer=on
  Delay1 : Delay  DelayLength=1  InitialCondition=0
  Gain : Gain  Gain=1/N
  Out : Outport
  wires:
  In/1 -> Delay/1, Add/2
  Gain/1 -> Out/1
  Delay/1 -> Add/3
  Add/1 -> Gain/1, Delay1/1
  Delay1/1 -> Add/1

== system quadripulse_controller16/Subsystem/Enabled Subsystem ==
  In1 : Inport
  Enable : EnablePort
  Buffer : Buffer  N=60*10  V=(60*10)-1  TreatMby1Signals=One channel  OutputFrames=off
  Out1 : Outport
  wires:
  In1/1 -> Buffer/1
  Buffer/1 -> Out1/1

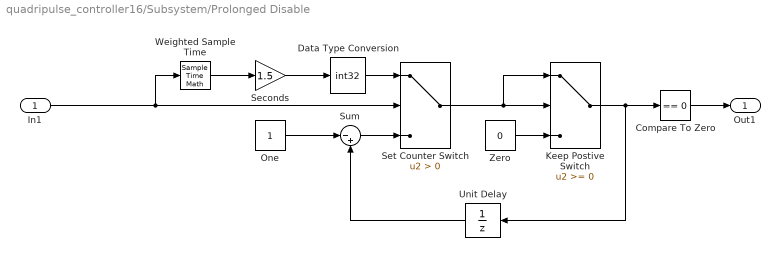
== system quadripulse_controller16/Subsystem/Prolonged Disable ==
  In1 : Inport
  Compare To Zero : simulink/Logic and Bit Operations/Compare To Zero  relop===  OutDataTypeStr=boolean
  Data Type Conversion : DataTypeConversion  OutDataTypeStr=int32
  Keep Postive Switch : Switch
  One : Constant  OutDataTypeStr=int32
  Seconds : Gain  Gain=1.5
  Set Counter Switch : Switch  Criteria=u2 > Threshold
  Sum : Sum  Inputs=|-+
  Unit Delay : UnitDelay  SampleTime=-1
  Weighted Sample Time : SampleTimeMath  TsampMathOp=1/Ts Only  weightValue=1
  Zero : Constant  Value=0  OutDataTypeStr=int32
  Out1 : Outport
  wires:
  One/1 -> Sum/1
  Compare To Zero/1 -> Out1/1
  Unit Delay/1 -> Sum/2
  Weighted Sample Time/1 -> Seconds/1
  Sum/1 -> Set Counter Switch/3
  Set Counter Switch/1 -> Keep Postive Switch/2, Keep Postive Switch/1
  Keep Postive Switch/1 -> Compare To Zero/1, Unit Delay/1
  Data Type Conversion/1 -> Set Counter Switch/1
  In1/1 -> Set Counter Switch/2, Weighted Sample Time/1
  Zero/1 -> Keep Postive Switch/3
  Seconds/1 -> Data Type Conversion/1

== system quadripulse_controller16/Time Series Forecast/Forecast of 128 samples ==
  Data : Inport
  Coefficients : Inport  Port=2
  Forecast : Subsystem
  Out1 : Outport
  wires:
  Forecast/1(Forecast) -> Out1/1
  Coefficients/1 -> Forecast/2(Coefficients)
  Data/1 -> Forecast/1(Vector)

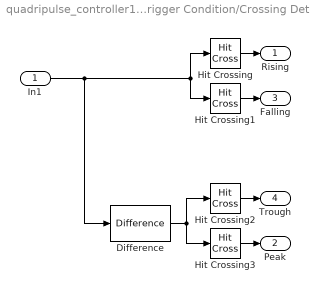
== system quadripulse_controller16/Trigger Condition/Crossing Detector ==
  In1 : Inport
  Difference : simulink/Discrete/Difference  ICPrevInput=0.0  InputProcessing=Inherited  OutMin=[]  OutMax=[]  OutDataType=fixdt(1, 16)  OutScaling=2^-10  DoSatur=off
  Hit Crossing : HitCross  HitCrossingDirection=rising
  Hit Crossing1 : HitCross  HitCrossingDirection=falling
  Hit Crossing2 : HitCross  HitCrossingDirection=rising
  Hit Crossing3 : HitCross  HitCrossingDirection=falling
  Rising : Outport
  Peak : Outport  Port=2
  Falling : Outport  Port=3
  Trough : Outport  Port=4
  wires:
  In1/1 -> Difference/1, Hit Crossing1/1, Hit Crossing/1
  Hit Crossing1/1 -> Falling/1
  Hit Crossing/1 -> Rising/1
  Difference/1 -> Hit Crossing3/1, Hit Crossing2/1
  Hit Crossing3/1 -> Peak/1
  Hit Crossing2/1 -> Trough/1

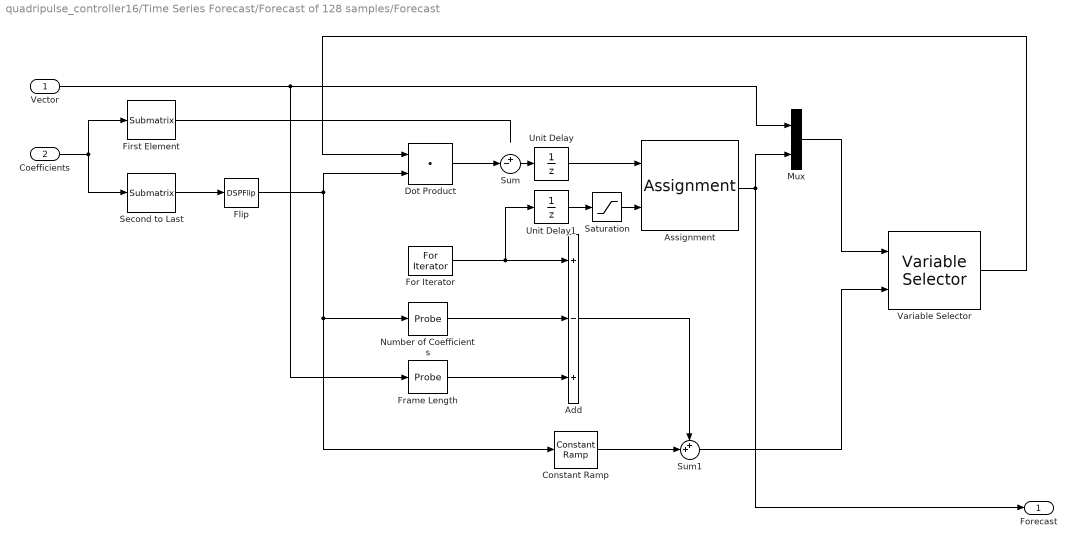
== system quadripulse_controller16/Time Series Forecast/Forecast of 128 samples/Forecast ==
  Vector : Inport
  Coefficients : Inport  Port=2
  Add : Sum  Inputs=+-+
  Assignment : Assignment  OutputInitialize=Specify size for each dimension in table  DiagnosticForDimensions=Warning  IndexOptions=Index vector (port)  Indices=1  OutputSizes=num_iterations
  Constant Ramp : dspsigops/Constant Ramp  L=Rows  dim=1  Slope=1  dataType=Same as input  isSigned=on  wordLen=16  udDataType=sfix(16)  fracBitsMode=Best precision  numFracBits=15  Offset=0
  Dot Product : DotProduct  InputSameDT=on  OutDataTypeStr=Inherit: Inherit via internal rule
  First Element : dspmtrx3/Submatrix  RowSpan=One row  RowStartMode=First  RowStartIndex=1  RowEndMode=Last  RowEndIndex=1  ColSpan=One column  ColStartMode=First  ColStartIndex=1  ColEndMode=Last  ColEndIndex=1
  Flip : DSPFlip
  For Iterator : ForIterator  IterationLimit=num_iterations+1
  Frame Length : Probe  ProbeSampleTime=off  ProbeComplexSignal=off
  Mux : Mux  Inputs=2
  Number of Coefficients : Probe  ProbeSampleTime=off  ProbeComplexSignal=off
  Saturation : Saturate  UpperLimit=num_iterations  LowerLimit=1
  Second to Last : dspmtrx3/Submatrix  RowSpan=Range of rows  RowStartMode=Index  RowStartIndex=2  RowEndMode=Last  RowEndIndex=1  ColSpan=One column  ColStartMode=First  ColStartIndex=1  ColEndMode=Last  ColEndIndex=1
  Sum : Sum  Inputs=+-|  OutDataTypeStr=double
  Sum1 : Sum  Inputs=++|  OutDataTypeStr=double
  Unit Delay : UnitDelay  SampleTime=-1
  Unit Delay1 : UnitDelay  SampleTime=-1
  Variable Selector : dspindex/Variable Selector  NumInputs=1  rowsOrCols=Rows  IdxMode=Variable  Elements=[1 3]  ZerOneIdxMode=One-based  errmode=Clip Index  FillMode=on  FillValues=0
  Forecast : Outport
  wires:
  Vector/1 -> Frame Length/1, Mux/1
  Mux/1 -> Variable Selector/1
  Assignment/1 -> Forecast/1, Mux/2
  Add/1 -> Sum1/1
  Frame Length/1 -> Add/3
  Number of Coefficients/1 -> Add/2
  Dot Product/1 -> Sum/2
  Constant Ramp/1 -> Sum1/2
  Sum1/1 -> Variable Selector/2
  Coefficients/1 -> First Element/1, Second to Last/1
  Second to Last/1 -> Flip/1
  Variable Selector/1 -> Dot Product/1
  Flip/1 -> Dot Product/2, Number of Coefficients/1, Constant Ramp/1
  First Element/1 -> ?
  Sum/1 -> Unit Delay/1
  For Iterator/1 -> Unit Delay1/1, Add/1
  Unit Delay/1 -> Assignment/1
  Unit Delay1/1 -> Saturation/1
  Saturation/1 -> Assignment/2
